simulink model "Saturation_Integrator"  (Simulink 7.5)
settings: Solver=ode45  StartTime=0.0  StopTime=10.0  RelTol=1e-3
settings Model: Creator=lm  LastModifiedBy=lm

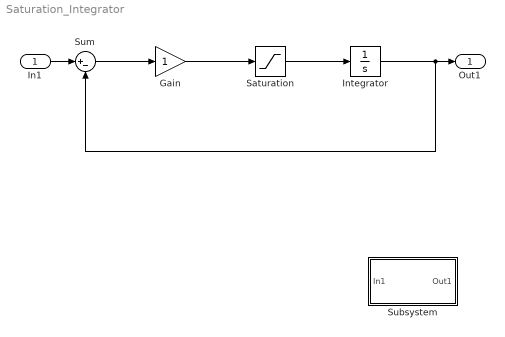
== system Saturation_Integrator ==
  In1 : Inport
  Gain : Gain  ParameterDataType=fixdt(1, 16)  ParameterScaling=2^0  OutDataType=fixdt(1, 16)  OutScaling=2^0
  Integrator : Integrator
  Saturation : Saturate  OutDataType=fixdt(1, 16)  OutScaling=2^0
  Subsystem : Subsystem
  Sum : Sum  Inputs=|+-  OutDataType=fixdt(1, 16)  OutScaling=2^0
  Out1 : Outport
  wires:
  Sum/1 -> Gain/1
  Gain/1 -> Saturation/1
  Saturation/1 -> Integrator/1
  Integrator/1 -> Out1/1, Sum/2
  In1/1 -> Sum/1

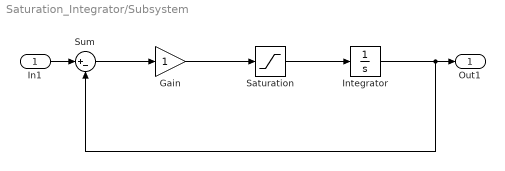
== system Saturation_Integrator/Subsystem ==
  In1 : Inport
  Gain : Gain  ParameterDataType=fixdt(1, 16)  ParameterScaling=2^0  OutDataType=fixdt(1, 16)  OutScaling=2^0
  Integrator : Integrator
  Saturation : Saturate  OutDataType=fixdt(1, 16)  OutScaling=2^0
  Sum : Sum  Inputs=|+-  OutDataType=fixdt(1, 16)  OutScaling=2^0
  Out1 : Outport
  wires:
  Sum/1 -> Gain/1
  Gain/1 -> Saturation/1
  Saturation/1 -> Integrator/1
  Integrator/1 -> Sum/2, Out1/1
  In1/1 -> Sum/1
